simulink model "ADCS"  (R2024a)
settings: Solver=FixedStepDiscrete  StartTime=0.0  StopTime=86400  FixedStep=1  RelTol=1e-3  EnableMultiTasking=on
undefined symbols (not defined in the file): deg, rad, s
libraries: aerolibconvert2 x4, sharedtransform x3, aerolibutil x2
settings Model: Creator=Abhishek  LastModifiedBy=Abhishek
settings SolverCC: AutoInsertRateTranBlk=on

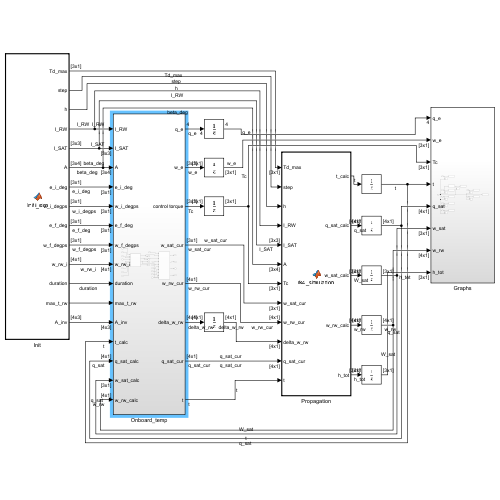
[thumbnail: Simulink's stored preview of the top-level diagram]
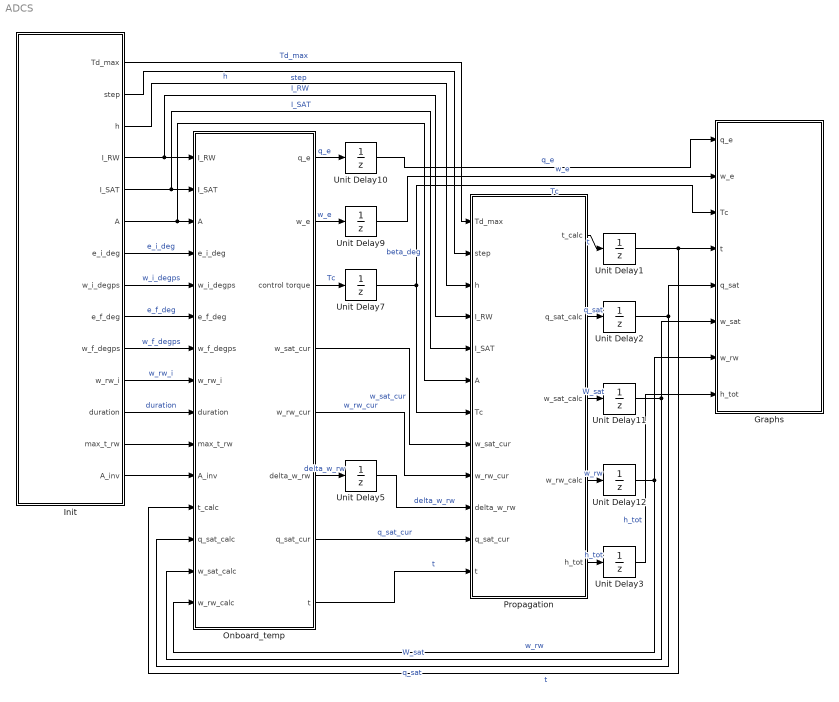
== system ADCS ==
  Graphs : Subsystem
  Init : MATLAB Function  TreatAsAtomicUnit=on
  Onboard_temp : Subsystem
  Propagation : MATLAB Function  TreatAsAtomicUnit=on
  Unit Delay{1..3,5,7,9..12} (9 alike) : UnitDelay  SampleTime=-1  HasFrameUpgradeWarning=on
  wires:
  Init/8(w_i_degps) -> Onboard_temp/5(w_i_degps)  "w_i_degps"
  Init/5(I_SAT) -> Onboard_temp/2(I_SAT), Propagation/5(I_SAT)  "I_SAT"
  Init/10(w_f_degps) -> Onboard_temp/7(w_f_degps)  "w_f_degps"
  Init/4(I_RW) -> Onboard_temp/1(I_RW), Propagation/4(I_RW)  "I_RW"
  Init/7(e_i_deg) -> Onboard_temp/4(e_i_deg)  "e_i_deg"
  Init/9(e_f_deg) -> Onboard_temp/6(e_f_deg)  "e_f_deg"
  Unit Delay11/1 -> Onboard_temp/14(w_sat_calc), Graphs/6(w_sat)  "W_sat"
  Init/2(step) -> Propagation/2(step)  "step"
  Init/11(w_rw_i) -> Onboard_temp/8(w_rw_i)  "w_rw_i"
  Init/3(h) -> Propagation/3(h)  "h"
  Init/12(duration) -> Onboard_temp/9(duration)  "duration"
  Unit Delay2/1 -> Onboard_temp/13(q_sat_calc), Graphs/5(q_sat)  "q_sat"
  Unit Delay9/1 -> Graphs/2(w_e)  "w_e"
  Init/6(A) -> Onboard_temp/3(A), Propagation/6(A)  "beta_deg"
  Unit Delay1/1 -> Graphs/4(t), Onboard_temp/12(t_calc)  "t"
  Init/1(Td_max) -> Propagation/1(Td_max)  "Td_max"
  Unit Delay7/1 -> Propagation/7(Tc), Graphs/3(Tc)  "Tc"
  Unit Delay10/1 -> Graphs/1(q_e)  "q_e"
  Unit Delay5/1 -> Propagation/10(delta_w_rw)  "delta_w_rw"
  Onboard_temp/8(t) -> Propagation/12(t)  "t"
  Onboard_temp/7(q_sat_cur) -> Propagation/11(q_sat_cur)  "q_sat_cur"
  Onboard_temp/6(delta_w_rw) -> Unit Delay5/1  "delta_w_rw"
  Onboard_temp/5(w_rw_cur) -> Propagation/9(w_rw_cur)  "w_rw_cur"
  Onboard_temp/3(control torque) -> Unit Delay7/1  "Tc"
  Onboard_temp/4(w_sat_cur) -> Propagation/8(w_sat_cur)  "w_sat_cur"
  Onboard_temp/2(w_e) -> Unit Delay9/1  "w_e"
  Onboard_temp/1(q_e) -> Unit Delay10/1  "q_e"
  Unit Delay12/1 -> Onboard_temp/15(w_rw_calc), Graphs/7(w_rw)  "w_rw"
  Propagation/1(t_calc) -> Unit Delay1/1  "t"
  Propagation/2(q_sat_calc) -> Unit Delay2/1  "q_sat"
  Propagation/3(w_sat_calc) -> Unit Delay11/1  "W_sat"
  Propagation/4(w_rw_calc) -> Unit Delay12/1  "w_rw"
  Init/14(A_inv) -> Onboard_temp/11(A_inv)
  Init/13(max_t_rw) -> Onboard_temp/10(max_t_rw)
  Unit Delay3/1 -> Graphs/8(h_tot)  "h_tot"
  Propagation/5(h_tot) -> Unit Delay3/1  "h_tot"

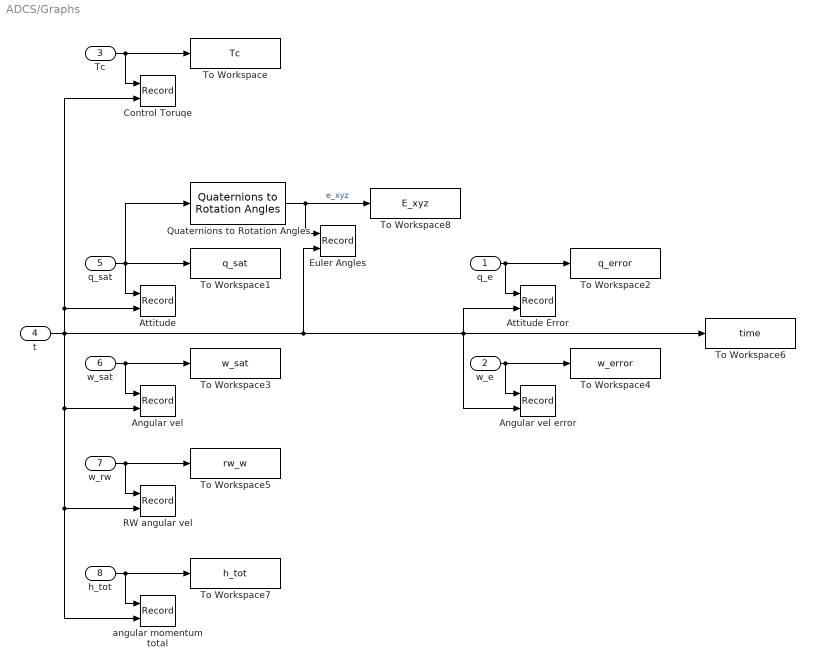
== system ADCS/Graphs ==
  q_e : Inport
  w_e : Inport  Port=2
  Tc : Inport  Port=3
  t : Inport  Port=4
  q_sat : Inport  Port=5
  w_sat : Inport  Port=6
  w_rw : Inport  Port=7
  h_tot : Inport  Port=8
  Angular vel : Record  FileSettingsInternal="{\"entries\":[{\"content\":{\"excelSettings\":{\"content\":{},\"type\":\"Streamout.ExcelSettings\"}},\"type\":\"Streamout.FileSettingStorage\",\"uuid\":\"\"}],\"packageUris\":[\"http:\\/\\/schema.mathworks.com\\/mf0\\/streamout_blocks\\/R2020a\"],\"version\":\"1.0\"}"  Layout=[1 1]  SignalsInternal="{\"entries\":[{\"content\":{\"signals\":[{\"content\":{\"blockPath\":[],\"dimensions\":[3,1],\"domain\":\"\",\"hasChildren\":true,\"lineColor\":\"#139fff\",\"lineWidth\":2,\"port\":1,\"sid\":[\"\"],\"signalID\":1,\"signalName\":\"w_sat\"},\"type\":\"RecordBlkView.Signal\",\"uuid\":\"\"},{\"content\":{\"blockPath\":[],\"channel\":[1,1],\"dimensions\":[3,1],\"domain\":\"\",\"lineColor\":\"#139fff\",\"lineWidth\":2,\"parentID\":1,\"plots\":[ 1 ],\"port\":1,\"sid\":[\"\"],\"signalID\":2,\"signalName\":\"w_sat\"},\"type\":\"RecordBlkView.Signal\",\"uuid\":\"\"},{\"content\":{\"blockPath\":[],\"dimensions\":[1],\"domain\":\"\",\"lineColor\":\"#ff6929\",\"lineWidth\":2,\"port\":2,\"sid\":[\"\"],\"signalID\":3,\"signalName\":\"t\"},\"type\":\"RecordBlkView.Signal\",\"uuid\":\"\"},{\"content\":{\"blockPath\":[],\"channel\":[2,1],\"dimensions\":[3,1],\"domain\":\"\",\"lineColor\":\"#4dbeee\",\"lineWidth\":2,\"parentID\":1,\"plots\":[ 1 ],\"port\":1,\"sid\":[\"\"],\"signalID\":4,\"signalName\":\"w_sat\"},\"type\":\"RecordBlkView.Signal\",\"uuid\":\"\"},{\"content\":{\"blockPath\":[],\"channel\":[3,1],\"dimensions\":[3,1],\"domain\":\"\",\"lineColor\":\"#a2142f\",\"lineWidth\":2,\"parentID\":1,\"plots\":[ 1 ],\"port\":1,\"sid\":[\"\"],\"signalID\":5,\"signalName\":\"w_sat\"},\"type\":\"RecordBlkView.Signal\",\"uuid\":\"\"}]},\"type\":\"RecordBlkView.InputSignals\",\"uuid\":\"\"}],\"packageUris\":[\"http:\\/\\/schema.mathworks.com\\/mf0\\/streamout_blocks\\/R2020a\"],\"version\":\"1.0\"}"  CompatibilityTag=XY
  Angular vel error : Record  FileSettingsInternal="{\"entries\":[{\"content\":{\"excelSettings\":{\"content\":{},\"type\":\"Streamout.ExcelSettings\"}},\"type\":\"Streamout.FileSettingStorage\",\"uuid\":\"\"}],\"packageUris\":[\"http:\\/\\/schema.mathworks.com\\/mf0\\/streamout_blocks\\/R2020a\"],\"version\":\"1.0\"}"  Layout=[1 1]  SignalsInternal="{\"entries\":[{\"content\":{\"signals\":[{\"content\":{\"blockPath\":[],\"dimensions\":[3,1],\"domain\":\"\",\"hasChildren\":true,\"lineColor\":\"#64d413\",\"lineWidth\":2,\"port\":1,\"sid\":[\"\"],\"signalID\":1,\"signalName\":\"w_e\"},\"type\":\"RecordBlkView.Signal\",\"uuid\":\"\"},{\"content\":{\"blockPath\":[],\"channel\":[1,1],\"dimensions\":[3,1],\"domain\":\"\",\"lineColor\":\"#64d413\",\"lineWidth\":2,\"parentID\":1,\"plots\":[ 1 ],\"port\":1,\"sid\":[\"\"],\"signalID\":2,\"signalName\":\"w_e\"},\"type\":\"RecordBlkView.Signal\",\"uuid\":\"\"},{\"content\":{\"blockPath\":[],\"dimensions\":[1],\"domain\":\"\",\"lineColor\":\"#ff13a6\",\"lineWidth\":2,\"port\":2,\"sid\":[\"\"],\"signalID\":3,\"signalName\":\"t\"},\"type\":\"RecordBlkView.Signal\",\"uuid\":\"\"},{\"content\":{\"blockPath\":[],\"channel\":[2,1],\"dimensions\":[3,1],\"domain\":\"\",\"lineColor\":\"#139fff\",\"lineWidth\":2,\"parentID\":1,\"plots\":[ 1 ],\"port\":1,\"sid\":[\"\"],\"signalID\":4,\"signalName\":\"w_e\"},\"type\":\"RecordBlkView.Signal\",\"uuid\":\"\"},{\"content\":{\"blockPath\":[],\"channel\":[3,1],\"dimensions\":[3,1],\"domain\":\"\",\"lineColor\":\"#ff6929\",\"lineWidth\":2,\"parentID\":1,\"plots\":[ 1 ],\"port\":1,\"sid\":[\"\"],\"signalID\":5,\"signalName\":\"w_e\"},\"type\":\"RecordBlkView.Signal\",\"uuid\":\"\"}]},\"type\":\"RecordBlkView.InputSignals\",\"uuid\":\"\"}],\"packageUris\":[\"http:\\/\\/schema.mathworks.com\\/mf0\\/streamout_blocks\\/R2020a\"],\"version\":\"1.0\"}"  CompatibilityTag=XY
  Attitude : Record  RecordToWorkspace=on  FileSettingsInternal="{\"entries\":[{\"content\":{\"excelSettings\":{\"content\":{},\"type\":\"Streamout.ExcelSettings\"}},\"type\":\"Streamout.FileSettingStorage\",\"uuid\":\"\"}],\"packageUris\":[\"http:\\/\\/schema.mathworks.com\\/mf0\\/streamout_blocks\\/R2020a\"],\"version\":\"1.0\"}"  Layout=[1 1]  SignalsInternal="{\"entries\":[{\"content\":{\"signals\":[{\"content\":{\"blockPath\":[],\"dimensions\":[4,1],\"domain\":\"\",\"hasChildren\":true,\"lineColor\":\"#22b573\",\"lineWidth\":2,\"port\":1,\"sid\":[\"\"],\"signalID\":1,\"signalName\":\"q_sat\"},\"type\":\"RecordBlkView.Signal\",\"uuid\":\"\"},{\"content\":{\"blockPath\":[],\"channel\":[1,1],\"dimensions\":[4,1],\"domain\":\"\",\"lineColor\":\"#22b573\",\"lineWidth\":2,\"parentID\":1,\"plots\":[ 1 ],\"port\":1,\"sid\":[\"\"],\"signalID\":2,\"signalName\":\"q_sat\"},\"type\":\"RecordBlkView.Signal\",\"uuid\":\"\"},{\"content\":{\"blockPath\":[],\"dimensions\":[1],\"domain\":\"\",\"lineColor\":\"#0072bd\",\"lineWidth\":2,\"port\":2,\"sid\":[\"\"],\"signalID\":3,\"signalName\":\"t\"},\"type\":\"RecordBlkView.Signal\",\"uuid\":\"\"},{\"content\":{\"blockPath\":[],\"channel\":[2,1],\"dimensions\":[4,1],\"domain\":\"\",\"lineColor\":\"#b746ff\",\"lineWidth\":2,\"parentID\":1,\"plots\":[ 1 ],\"port\":1,\"sid\":[\"\"],\"signalID\":4,\"signalName\":\"q_sat\"},\"type\":\"RecordBlkView.Signal\",\"uuid\":\"\"},{\"content\":{\"blockPath\":[],\"channel\":[3,1],\"dimensions\":[4,1],\"domain\":\"\",\"lineColor\":\"#64d413\",\"lineWidth\":2,\"parentID\":1,\"plots\":[ 1 ],\"port\":1,\"sid\":[\"\"],\"signalID\":5,\"signalName\":\"q_sat\"},\"type\":\"RecordBlkView.Signal\",\"uuid\":\"\"},{\"content\":{\"blockPath\":[],\"channel\":[4,1],\"dimensions\":[4,1],\"domain\":\"\",\"lineColor\":\"#ff13a6\",\"lineWidth\":2,\"parentID\":1,\"plots\":[ 1 ],\"port\":1,\"sid\":[\"\"],\"signalID\":6,\"signalName\":\"q_sat\"},\"type\":\"RecordBlkView.Signal\",\"uuid\":\"\"}]},\"type\":\"RecordBlkView.InputSignals\",\"uuid\":\"\"}],\"packageUris\":[\"http:\\/\\/schema.mathworks.com\\/mf0\\/streamout_blocks\\/R2020a\"],\"version\":\"1.0\"}"  CompatibilityTag=XY
  Attitude Error : Record  FileSettingsInternal="{\"entries\":[{\"content\":{\"excelSettings\":{\"content\":{},\"type\":\"Streamout.ExcelSettings\"}},\"type\":\"Streamout.FileSettingStorage\",\"uuid\":\"\"}],\"packageUris\":[\"http:\\/\\/schema.mathworks.com\\/mf0\\/streamout_blocks\\/R2020a\"],\"version\":\"1.0\"}"  Layout=[1 1]  SignalsInternal="{\"entries\":[{\"content\":{\"signals\":[{\"content\":{\"blockPath\":[],\"dimensions\":[4],\"domain\":\"\",\"hasChildren\":true,\"lineColor\":\"#edb120\",\"lineWidth\":2,\"port\":1,\"sid\":[\"\"],\"signalID\":1,\"signalName\":\"q_e\"},\"type\":\"RecordBlkView.Signal\",\"uuid\":\"\"},{\"content\":{\"blockPath\":[],\"channel\":[1],\"dimensions\":[4],\"domain\":\"\",\"lineColor\":\"#edb120\",\"lineWidth\":2,\"parentID\":1,\"plots\":[ 1 ],\"port\":1,\"sid\":[\"\"],\"signalID\":2,\"signalName\":\"q_e\"},\"type\":\"RecordBlkView.Signal\",\"uuid\":\"\"},{\"content\":{\"blockPath\":[],\"dimensions\":[1],\"domain\":\"\",\"lineColor\":\"#7e2f8e\",\"lineWidth\":2,\"port\":2,\"sid\":[\"\"],\"signalID\":3,\"signalName\":\"t\"},\"type\":\"RecordBlkView.Signal\",\"uuid\":\"\"},{\"content\":{\"blockPath\":[],\"channel\":[2],\"dimensions\":[4],\"domain\":\"\",\"lineColor\":\"#fe330a\",\"lineWidth\":2,\"parentID\":1,\"plots\":[ 1 ],\"port\":1,\"sid\":[\"\"],\"signalID\":4,\"signalName\":\"q_e\"},\"type\":\"RecordBlkView.Signal\",\"uuid\":\"\"},{\"content\":{\"blockPath\":[],\"channel\":[3],\"dimensions\":[4],\"domain\":\"\",\"lineColor\":\"#22b573\",\"lineWidth\":2,\"parentID\":1,\"plots\":[ 1 ],\"port\":1,\"sid\":[\"\"],\"signalID\":5,\"signalName\":\"q_e\"},\"type\":\"RecordBlkView.Signal\",\"uuid\":\"\"},{\"content\":{\"blockPath\":[],\"channel\":[4],\"dimensions\":[4],\"domain\":\"\",\"lineColor\":\"#0072bd\",\"lineWidth\":2,\"parentID\":1,\"plots\":[ 1 ],\"port\":1,\"sid\":[\"\"],\"signalID\":6,\"signalName\":\"q_e\"},\"type\":\"RecordBlkView.Signal\",\"uuid\":\"\"}]},\"type\":\"RecordBlkView.InputSignals\",\"uuid\":\"\"}],\"packageUris\":[\"http:\\/\\/schema.mathworks.com\\/mf0\\/streamout_blocks\\/R2020a\"],\"version\":\"1.0\"}"  CompatibilityTag=XY
  Control Toruqe : Record  FileSettingsInternal="{\"entries\":[{\"content\":{\"excelSettings\":{\"content\":{},\"type\":\"Streamout.ExcelSettings\"}},\"type\":\"Streamout.FileSettingStorage\",\"uuid\":\"\"}],\"packageUris\":[\"http:\\/\\/schema.mathworks.com\\/mf0\\/streamout_blocks\\/R2020a\"],\"version\":\"1.0\"}"  Layout=[1 1]  SignalsInternal="{\"entries\":[{\"content\":{\"signals\":[{\"content\":{\"blockPath\":[],\"dimensions\":[3,1],\"domain\":\"\",\"hasChildren\":true,\"lineColor\":\"#4dbeee\",\"lineWidth\":2,\"port\":1,\"sid\":[\"\"],\"signalID\":1,\"signalName\":\"Tc\"},\"type\":\"RecordBlkView.Signal\",\"uuid\":\"\"},{\"content\":{\"blockPath\":[],\"channel\":[1,1],\"dimensions\":[3,1],\"domain\":\"\",\"lineColor\":\"#4dbeee\",\"lineWidth\":2,\"parentID\":1,\"plots\":[ 1 ],\"port\":1,\"sid\":[\"\"],\"signalID\":2,\"signalName\":\"Tc\"},\"type\":\"RecordBlkView.Signal\",\"uuid\":\"\"},{\"content\":{\"blockPath\":[],\"dimensions\":[1],\"domain\":\"\",\"lineColor\":\"#a2142f\",\"lineWidth\":2,\"port\":2,\"sid\":[\"\"],\"signalID\":3,\"signalName\":\"t\"},\"type\":\"RecordBlkView.Signal\",\"uuid\":\"\"},{\"content\":{\"blockPath\":[],\"channel\":[2,1],\"dimensions\":[3,1],\"domain\":\"\",\"lineColor\":\"#d95319\",\"lineWidth\":2,\"parentID\":1,\"plots\":[ 1 ],\"port\":1,\"sid\":[\"\"],\"signalID\":4,\"signalName\":\"Tc\"},\"type\":\"RecordBlkView.Signal\",\"uuid\":\"\"},{\"content\":{\"blockPath\":[],\"channel\":[3,1],\"dimensions\":[3,1],\"domain\":\"\",\"lineColor\":\"#edb120\",\"lineWidth\":2,\"parentID\":1,\"plots\":[ 1 ],\"port\":1,\"sid\":[\"\"],\"signalID\":5,\"signalName\":\"Tc\"},\"type\":\"RecordBlkView.Signal\",\"uuid\":\"\"}]},\"type\":\"RecordBlkView.InputSignals\",\"uuid\":\"\"}],\"packageUris\":[\"http:\\/\\/schema.mathworks.com\\/mf0\\/streamout_blocks\\/R2020a\"],\"version\":\"1.0\"}"  CompatibilityTag=XY
  Euler Angles : Record  FileSettingsInternal="{\"entries\":[{\"content\":{\"excelSettings\":{\"content\":{},\"type\":\"Streamout.ExcelSettings\"}},\"type\":\"Streamout.FileSettingStorage\",\"uuid\":\"\"}],\"packageUris\":[\"http:\\/\\/schema.mathworks.com\\/mf0\\/streamout_blocks\\/R2020a\"],\"version\":\"1.0\"}"  Layout=[1 1]  SignalsInternal="{\"entries\":[{\"content\":{\"signals\":[{\"content\":{\"blockPath\":[],\"dimensions\":[3],\"domain\":\"\",\"hasChildren\":true,\"lineColor\":\"#ff6929\",\"lineWidth\":2,\"port\":1,\"sid\":[\"\"],\"signalID\":1,\"signalName\":\"e_xyz\"},\"type\":\"RecordBlkView.Signal\",\"uuid\":\"\"},{\"content\":{\"blockPath\":[],\"channel\":[1],\"dimensions\":[3],\"domain\":\"\",\"lineColor\":\"#ff6929\",\"lineWidth\":2,\"parentID\":1,\"plots\":[ 1 ],\"port\":1,\"sid\":[\"\"],\"signalID\":2,\"signalName\":\"e_xyz\"},\"type\":\"RecordBlkView.Signal\",\"uuid\":\"\"},{\"content\":{\"blockPath\":[],\"dimensions\":[1],\"domain\":\"\",\"lineColor\":\"#b746ff\",\"lineWidth\":2,\"port\":2,\"sid\":[\"\"],\"signalID\":3,\"signalName\":\"t\"},\"type\":\"RecordBlkView.Signal\",\"uuid\":\"\"},{\"content\":{\"blockPath\":[],\"channel\":[2],\"dimensions\":[3],\"domain\":\"\",\"lineColor\":\"#7e2f8e\",\"lineWidth\":2,\"parentID\":1,\"plots\":[ 1 ],\"port\":1,\"sid\":[\"\"],\"signalID\":4,\"signalName\":\"e_xyz\"},\"type\":\"RecordBlkView.Signal\",\"uuid\":\"\"},{\"content\":{\"blockPath\":[],\"channel\":[3],\"dimensions\":[3],\"domain\":\"\",\"lineColor\":\"#77ac30\",\"lineWidth\":2,\"parentID\":1,\"plots\":[ 1 ],\"port\":1,\"sid\":[\"\"],\"signalID\":5,\"signalName\":\"e_xyz\"},\"type\":\"RecordBlkView.Signal\",\"uuid\":\"\"}]},\"type\":\"RecordBlkView.InputSignals\",\"uuid\":\"\"}],\"packageUris\":[\"http:\\/\\/schema.mathworks.com\\/mf0\\/streamout_blocks\\/R2020a\"],\"version\":\"1.0\"}"  CompatibilityTag=XY
  Quaternions to Rotation Angles : sharedtransform/Quaternions to Rotation Angles  rotationOrder=XYZ  aMode=aMode
  RW angular vel : Record  FileSettingsInternal="{\"entries\":[{\"content\":{\"excelSettings\":{\"content\":{},\"type\":\"Streamout.ExcelSettings\"}},\"type\":\"Streamout.FileSettingStorage\",\"uuid\":\"\"}],\"packageUris\":[\"http:\\/\\/schema.mathworks.com\\/mf0\\/streamout_blocks\\/R2020a\"],\"version\":\"1.0\"}"  Layout=[1 1]  SignalsInternal="{\"entries\":[{\"content\":{\"signals\":[{\"content\":{\"blockPath\":[],\"dimensions\":[4,1],\"domain\":\"\",\"hasChildren\":true,\"lineColor\":\"#ff13a6\",\"lineWidth\":2,\"port\":1,\"sid\":[\"\"],\"signalID\":1,\"signalName\":\"w_rw\"},\"type\":\"RecordBlkView.Signal\",\"uuid\":\"\"},{\"content\":{\"blockPath\":[],\"channel\":[1,1],\"dimensions\":[4,1],\"domain\":\"\",\"lineColor\":\"#ff13a6\",\"lineWidth\":2,\"parentID\":1,\"plots\":[ 1 ],\"port\":1,\"sid\":[\"\"],\"signalID\":2,\"signalName\":\"w_rw\"},\"type\":\"RecordBlkView.Signal\",\"uuid\":\"\"},{\"content\":{\"blockPath\":[],\"dimensions\":[1],\"domain\":\"\",\"lineColor\":\"#fe330a\",\"lineWidth\":2,\"port\":2,\"sid\":[\"\"],\"signalID\":3,\"signalName\":\"t\"},\"type\":\"RecordBlkView.Signal\",\"uuid\":\"\"},{\"content\":{\"blockPath\":[],\"channel\":[2,1],\"dimensions\":[4,1],\"domain\":\"\",\"lineColor\":\"#4dbeee\",\"lineWidth\":2,\"parentID\":1,\"plots\":[ 1 ],\"port\":1,\"sid\":[\"\"],\"signalID\":4,\"signalName\":\"w_rw\"},\"type\":\"RecordBlkView.Signal\",\"uuid\":\"\"},{\"content\":{\"blockPath\":[],\"channel\":[3,1],\"dimensions\":[4,1],\"domain\":\"\",\"lineColor\":\"#a2142f\",\"lineWidth\":2,\"parentID\":1,\"plots\":[ 1 ],\"port\":1,\"sid\":[\"\"],\"signalID\":5,\"signalName\":\"w_rw\"},\"type\":\"RecordBlkView.Signal\",\"uuid\":\"\"},{\"content\":{\"blockPath\":[],\"channel\":[4,1],\"dimensions\":[4,1],\"domain\":\"\",\"lineColor\":\"#139fff\",\"lineWidth\":2,\"parentID\":1,\"plots\":[ 1 ],\"port\":1,\"sid\":[\"\"],\"signalID\":6,\"signalName\":\"w_rw\"},\"type\":\"RecordBlkView.Signal\",\"uuid\":\"\"}]},\"type\":\"RecordBlkView.InputSignals\",\"uuid\":\"\"}],\"packageUris\":[\"http:\\/\\/schema.mathworks.com\\/mf0\\/streamout_blocks\\/R2020a\"],\"version\":\"1.0\"}"  CompatibilityTag=XY
  To Workspace : ToWorkspace  VariableName=Tc  SampleTime=-1
  To Workspace1 : ToWorkspace  VariableName=q_sat  SampleTime=-1
  To Workspace2 : ToWorkspace  VariableName=q_error  SampleTime=-1
  To Workspace3 : ToWorkspace  VariableName=w_sat  SampleTime=-1
  To Workspace4 : ToWorkspace  VariableName=w_error  SampleTime=-1
  To Workspace5 : ToWorkspace  VariableName=rw_w  SampleTime=-1
  To Workspace6 : ToWorkspace  VariableName=time  SampleTime=-1
  To Workspace7 : ToWorkspace  VariableName=h_tot  SampleTime=-1
  To Workspace8 : ToWorkspace  VariableName=E_xyz  SampleTime=-1
  angular momentum total : Record  FileSettingsInternal="{\"entries\":[{\"content\":{\"excelSettings\":{\"content\":{},\"type\":\"Streamout.ExcelSettings\"}},\"type\":\"Streamout.FileSettingStorage\",\"uuid\":\"\"}],\"packageUris\":[\"http:\\/\\/schema.mathworks.com\\/mf0\\/streamout_blocks\\/R2020a\"],\"version\":\"1.0\"}"  Layout=[1 1]  SignalsInternal="{\"entries\":[{\"content\":{\"signals\":[{\"content\":{\"blockPath\":[],\"dimensions\":[3,1],\"domain\":\"\",\"hasChildren\":true,\"lineColor\":\"#7e2f8e\",\"lineWidth\":2,\"port\":1,\"sid\":[\"\"],\"signalID\":1,\"signalName\":\"h_tot\"},\"type\":\"RecordBlkView.Signal\",\"uuid\":\"\"},{\"content\":{\"blockPath\":[],\"channel\":[1,1],\"dimensions\":[3,1],\"domain\":\"\",\"lineColor\":\"#7e2f8e\",\"lineWidth\":2,\"parentID\":1,\"plots\":[ 1 ],\"port\":1,\"sid\":[\"\"],\"signalID\":2,\"signalName\":\"h_tot\"},\"type\":\"RecordBlkView.Signal\",\"uuid\":\"\"},{\"content\":{\"blockPath\":[],\"dimensions\":[1],\"domain\":\"\",\"lineColor\":\"#77ac30\",\"lineWidth\":2,\"port\":2,\"sid\":[\"\"],\"signalID\":3,\"signalName\":\"t\"},\"type\":\"RecordBlkView.Signal\",\"uuid\":\"\"},{\"content\":{\"blockPath\":[],\"channel\":[2,1],\"dimensions\":[3,1],\"domain\":\"\",\"lineColor\":\"#22b573\",\"lineWidth\":2,\"parentID\":1,\"plots\":[ 1 ],\"port\":1,\"sid\":[\"\"],\"signalID\":4,\"signalName\":\"h_tot\"},\"type\":\"RecordBlkView.Signal\",\"uuid\":\"\"},{\"content\":{\"blockPath\":[],\"channel\":[3,1],\"dimensions\":[3,1],\"domain\":\"\",\"lineColor\":\"#0072bd\",\"lineWidth\":2,\"parentID\":1,\"plots\":[ 1 ],\"port\":1,\"sid\":[\"\"],\"signalID\":5,\"signalName\":\"h_tot\"},\"type\":\"RecordBlkView.Signal\",\"uuid\":\"\"}]},\"type\":\"RecordBlkView.InputSignals\",\"uuid\":\"\"}],\"packageUris\":[\"http:\\/\\/schema.mathworks.com\\/mf0\\/streamout_blocks\\/R2020a\"],\"version\":\"1.0\"}"  VisualizationBindings="{\"sparklinesplugin\":{\"info\":[{\"bindingParametersList\":[],\"subplotID\":1}]}}"  CompatibilityTag=XY
  wires:
  w_sat/1 -> To Workspace3/1, Angular vel/1
  q_e/1 -> Attitude Error/1, To Workspace2/1
  q_sat/1 -> To Workspace1/1, Quaternions to Rotation Angles/1, Attitude/1
  w_e/1 -> To Workspace4/1, Angular vel error/1
  Tc/1 -> To Workspace/1, Control Toruqe/1
  w_rw/1 -> RW angular vel/1, To Workspace5/1
  t/1 -> Euler Angles/2, To Workspace6/1, Attitude Error/2, Angular vel error/2, Angular vel/2, angular momentum total/2, RW angular vel/2, Attitude/2, Control Toruqe/2
  h_tot/1 -> To Workspace7/1, angular momentum total/1
  Quaternions to Rotation Angles/1 -> To Workspace8/1, Euler Angles/1  "e_xyz"

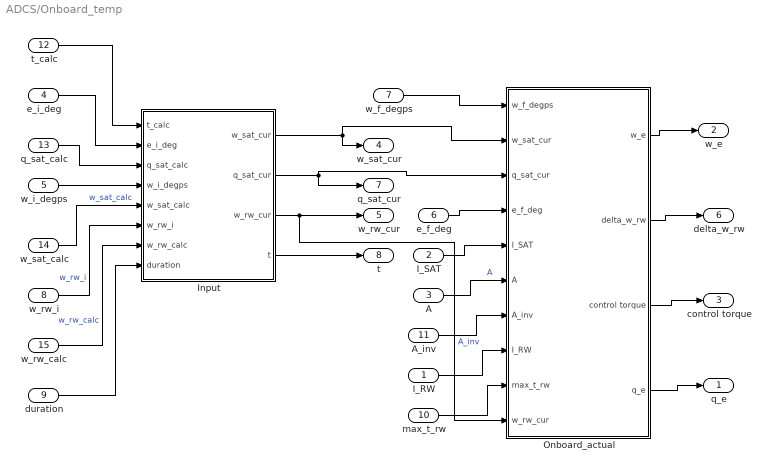
== system ADCS/Onboard_temp ==
  I_RW : Inport
  I_SAT : Inport  Port=2
  A : Inport  Port=3
  e_i_deg : Inport  Port=4
  w_i_degps : Inport  Port=5
  e_f_deg : Inport  Port=6
  w_f_degps : Inport  Port=7
  w_rw_i : Inport  Port=8
  duration : Inport  Port=9
  max_t_rw : Inport  Port=10
  A_inv : Inport  Port=11
  t_calc : Inport  Port=12
  q_sat_calc : Inport  Port=13
  w_sat_calc : Inport  Port=14
  w_rw_calc : Inport  Port=15
  Input : Subsystem
  Onboard_actual : Subsystem
  q_e : Outport
  w_e : Outport  Port=2
  control torque : Outport  Port=3
  w_sat_cur : Outport  Port=4
  w_rw_cur : Outport  Port=5
  delta_w_rw : Outport  Port=6
  q_sat_cur : Outport  Port=7
  t : Outport  Port=8
  wires:
  w_rw_i/1 -> Input/6(w_rw_i)  "w_rw_i"
  duration/1 -> Input/8(duration)
  Input/3(w_rw_cur) -> Onboard_actual/10(w_rw_cur), w_rw_cur/1
  w_rw_calc/1 -> Input/7(w_rw_calc)  "w_rw_calc"
  t_calc/1 -> Input/1(t_calc)
  Onboard_actual/1(w_e) -> w_e/1
  e_i_deg/1 -> Input/2(e_i_deg)
  q_sat_calc/1 -> Input/3(q_sat_calc)
  w_i_degps/1 -> Input/4(w_i_degps)
  w_sat_calc/1 -> Input/5(w_sat_calc)  "w_sat_calc"
  Input/1(w_sat_cur) -> w_sat_cur/1, Onboard_actual/2(w_sat_cur)
  Onboard_actual/3(control torque) -> control torque/1
  Input/2(q_sat_cur) -> q_sat_cur/1, Onboard_actual/3(q_sat_cur)
  Input/4(t) -> t/1
  w_f_degps/1 -> Onboard_actual/1(w_f_degps)
  e_f_deg/1 -> Onboard_actual/4(e_f_deg)
  I_SAT/1 -> Onboard_actual/5(I_SAT)
  Onboard_actual/2(delta_w_rw) -> delta_w_rw/1
  Onboard_actual/4(q_e) -> q_e/1
  A/1 -> Onboard_actual/6(A)  "A"
  I_RW/1 -> Onboard_actual/8(I_RW)
  A_inv/1 -> Onboard_actual/7(A_inv)  "A_inv"
  max_t_rw/1 -> Onboard_actual/9(max_t_rw)

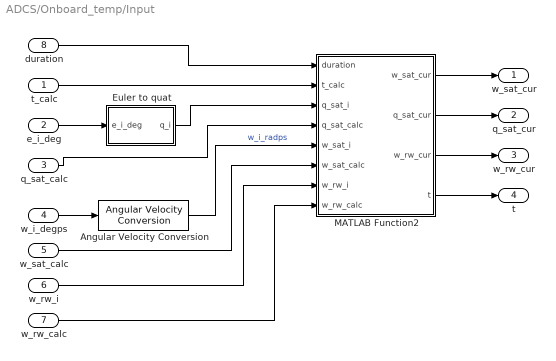
== system ADCS/Onboard_temp/Input ==
  t_calc : Inport
  e_i_deg : Inport  Port=2
  q_sat_calc : Inport  Port=3
  w_i_degps : Inport  Port=4
  w_sat_calc : Inport  Port=5
  w_rw_i : Inport  Port=6
  w_rw_calc : Inport  Port=7
  duration : Inport  Port=8
  Angular Velocity Conversion : aerolibconvert2/Angular Velocity Conversion  IU=deg/s  OU=rad/s
  Euler to quat : Subsystem
  MATLAB Function2 : MATLAB Function  TreatAsAtomicUnit=on
  w_sat_cur : Outport
  q_sat_cur : Outport  Port=2
  w_rw_cur : Outport  Port=3
  t : Outport  Port=4
  wires:
  MATLAB Function2/3(w_rw_cur) -> w_rw_cur/1
  Angular Velocity Conversion/1 -> MATLAB Function2/5(w_sat_i)  "w_i_radps"
  w_rw_calc/1 -> MATLAB Function2/8(w_rw_calc)
  MATLAB Function2/2(q_sat_cur) -> q_sat_cur/1
  Euler to quat/1(q_i) -> MATLAB Function2/3(q_sat_i)
  t_calc/1 -> MATLAB Function2/2(t_calc)
  w_i_degps/1 -> Angular Velocity Conversion/1
  q_sat_calc/1 -> MATLAB Function2/4(q_sat_calc)
  w_sat_calc/1 -> MATLAB Function2/6(w_sat_calc)
  w_rw_i/1 -> MATLAB Function2/7(w_rw_i)
  MATLAB Function2/4(t) -> t/1
  e_i_deg/1 -> Euler to quat/1(e_i_deg)
  MATLAB Function2/1(w_sat_cur) -> w_sat_cur/1
  duration/1 -> MATLAB Function2/1(duration)

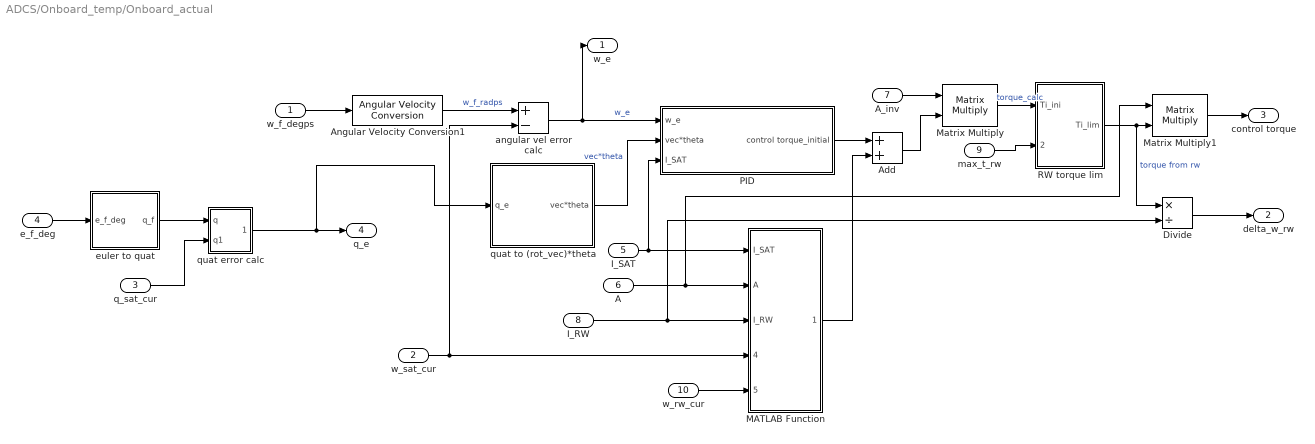
== system ADCS/Onboard_temp/Onboard_actual ==
  w_f_degps : Inport
  w_sat_cur : Inport  Port=2
  q_sat_cur : Inport  Port=3
  e_f_deg : Inport  Port=4
  I_SAT : Inport  Port=5
  A : Inport  Port=6
  A_inv : Inport  Port=7
  I_RW : Inport  Port=8
  max_t_rw : Inport  Port=9
  w_rw_cur : Inport  Port=10
  Add : Sum
  Angular Velocity Conversion1 : aerolibconvert2/Angular Velocity Conversion  IU=deg/s  OU=rad/s
  Divide : Product  Inputs=*/
  MATLAB Function : MATLAB Function  TreatAsAtomicUnit=on
  Matrix Multiply : Product  Multiplication=Matrix(*)
  Matrix Multiply1 : Product  Multiplication=Matrix(*)
  PID : Subsystem
  RW torque lim : MATLAB Function  TreatAsAtomicUnit=on
  angular vel error calc : Sum  Inputs=+-
  euler to quat : Subsystem
  quat error calc : Subsystem
  "quat to (rot_vec)*theta " : Subsystem
  w_e : Outport
  delta_w_rw : Outport  Port=2
  control torque : Outport  Port=3
  q_e : Outport  Port=4
  wires:
  Angular Velocity Conversion1/1 -> angular vel error calc/1  "w_f_radps"
  A_inv/1 -> Matrix Multiply/1
  q_sat_cur/1 -> quat error calc/2(q1)
  I_RW/1 -> MATLAB Function/3(I_RW), Divide/2
  e_f_deg/1 -> euler to quat/1(e_f_deg)
  quat error calc/1(q_e) -> "quat to (rot_vec)*theta "/1(q_e), q_e/1
  "quat to (rot_vec)*theta "/1(vec*theta) -> PID/2(vec*theta)  "vec*theta"
  w_sat_cur/1 -> MATLAB Function/4(w_sat_cur), angular vel error calc/2
  w_f_degps/1 -> Angular Velocity Conversion1/1
  angular vel error calc/1 -> w_e/1, PID/1(w_e)  "w_e"
  euler to quat/1(q_f) -> quat error calc/1(q)
  max_t_rw/1 -> RW torque lim/2(max_t_rw)
  I_SAT/1 -> MATLAB Function/1(I_SAT), PID/3(I_SAT)
  A/1 -> Matrix Multiply1/1, MATLAB Function/2(A)
  PID/1(control torque_initial) -> Add/1
  w_rw_cur/1 -> MATLAB Function/5(w_rw_cur)
  MATLAB Function/1(offset_Tc) -> Add/2
  Add/1 -> Matrix Multiply/2
  Matrix Multiply/1 -> RW torque lim/1(Ti_ini)  "torque_calc"
  RW torque lim/1(Ti_lim) -> Divide/1, Matrix Multiply1/2  "torque from rw"
  Matrix Multiply1/1 -> control torque/1
  Divide/1 -> delta_w_rw/1

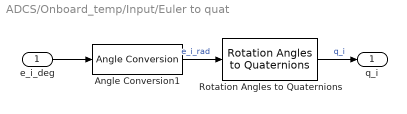
== system ADCS/Onboard_temp/Input/Euler to quat ==
  e_i_deg : Inport
  Angle Conversion1 : aerolibconvert2/Angle Conversion  IU=deg  OU=rad
  Rotation Angles to Quaternions : sharedtransform/Rotation Angles to Quaternions  rotationOrder=XYZ  aMode=aMode
  q_i : Outport
  wires:
  e_i_deg/1 -> Angle Conversion1/1
  Rotation Angles to Quaternions/1 -> q_i/1  "q_i"
  Angle Conversion1/1 -> Rotation Angles to Quaternions/1  "e_i_rad"

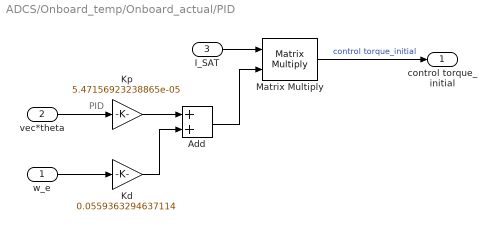
== system ADCS/Onboard_temp/Onboard_actual/PID ==
  note: PID
  w_e : Inport
  vec*theta : Inport  Port=2
  I_SAT : Inport  Port=3
  Add : Sum
  Kd : Gain  Gain=0.0559363294637114
  Kp : Gain  Gain=5.47156923238865e-05
  Matrix Multiply : Product  Multiplication=Matrix(*)
  control torque_initial : Outport
  wires:
  Matrix Multiply/1 -> control torque_initial/1  "control torque_initial"
  Kd/1 -> Add/2
  Kp/1 -> Add/1
  I_SAT/1 -> Matrix Multiply/1
  w_e/1 -> Kd/1
  vec*theta/1 -> Kp/1
  Add/1 -> Matrix Multiply/2

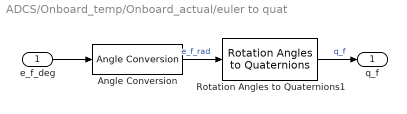
== system ADCS/Onboard_temp/Onboard_actual/euler to quat ==
  e_f_deg : Inport
  Angle Conversion : aerolibconvert2/Angle Conversion  IU=deg  OU=rad
  Rotation Angles to Quaternions1 : sharedtransform/Rotation Angles to Quaternions  rotationOrder=XYZ  aMode=aMode
  q_f : Outport
  wires:
  e_f_deg/1 -> Angle Conversion/1
  Angle Conversion/1 -> Rotation Angles to Quaternions1/1  "e_f_rad"
  Rotation Angles to Quaternions1/1 -> q_f/1  "q_f"

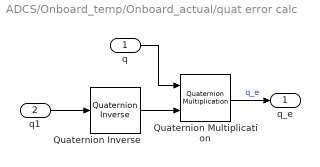
== system ADCS/Onboard_temp/Onboard_actual/quat error calc ==
  q : Inport
  q1 : Inport  Port=2
  Quaternion Inverse : aerolibutil/Quaternion Inverse
  Quaternion Multiplication : aerolibutil/Quaternion Multiplication
  q_e : Outport
  wires:
  q/1 -> Quaternion Multiplication/1
  q1/1 -> Quaternion Inverse/1
  Quaternion Multiplication/1 -> q_e/1  "q_e"
  Quaternion Inverse/1 -> Quaternion Multiplication/2

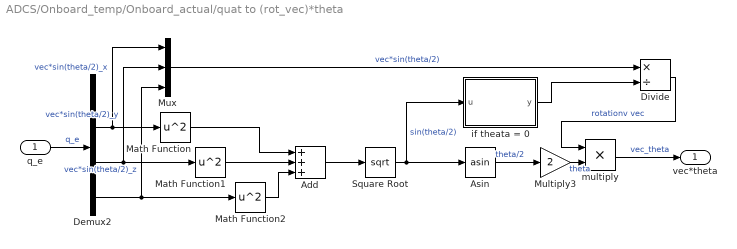
== system ADCS/Onboard_temp/Onboard_actual/quat to (rot_vec)*theta  ==
  q_e : Inport
  Add : Sum  Inputs=+++
  Asin : Trigonometry  Operator=asin
  Demux2 : Demux
  Divide : Product  Inputs=*/
  Math Function : Math  Operator=square
  Math Function1 : Math  Operator=square
  Math Function2 : Math  Operator=square
  Multiply3 : Gain  Gain=2
  Mux : Mux  Inputs=3
  Square Root : Sqrt
  if theata = 0 : MATLAB Function  TreatAsAtomicUnit=on
  multiply : Product  Inputs=**
  vec*theta : Outport
  wires:
  Demux2/2 -> Math Function/1, Mux/1  "vec*sin(theta/2)_x"
  Math Function2/1 -> Add/3
  Demux2/3 -> Math Function1/1, Mux/2  "vec*sin(theta/2)_y"
  Demux2/4 -> Math Function2/1, Mux/3  "vec*sin(theta/2)_z"
  Math Function1/1 -> Add/2
  q_e/1 -> Demux2/1  "q_e"
  Math Function/1 -> Add/1
  Add/1 -> Square Root/1
  Square Root/1 -> if theata = 0/1(u), Asin/1  "sin(theta/2)"
  Divide/1 -> multiply/1  "rotationv vec"
  Asin/1 -> Multiply3/1  "theta/2"
  Multiply3/1 -> multiply/2  "theta"
  multiply/1 -> vec*theta/1  "vec_theta"
  Mux/1 -> Divide/1  "vec*sin(theta/2)"
  if theata = 0/1(y) -> Divide/2

== matlab function ADCS/Onboard_temp/Onboard_actual/quat to (rot_vec)*theta /if theata = 0 ==
  data: u input; y output
function y = checking_zero(u)
    y=u;
    if u==0.00;
        y=1.00;
    end
end

== matlab function ADCS/Onboard_temp/Onboard_actual/MATLAB Function ==
  data: I_SAT input; A input; offset_Tc output; I_RW input; w_sat_cur input; w_rw_cur input
function offset_Tc = fcn(I_SAT,A,I_RW,w_sat_cur, w_rw_cur)
    offset_Tc=[0;0;0];
    H_sat= I_SAT*w_sat_cur;
    H_rw= A*(I_RW*w_rw_cur);
    offset_Tc=cross(w_sat_cur,H_sat)+cross(w_sat_cur,H_rw); 
end

== matlab function ADCS/Init ==
  data: Td_max output; step output; h output; I_RW output; I_SAT output; A output; e_i_deg output; w_i_degps output; e_f_deg output; w_f_degps output; w_rw_i output; duration output; max_t_rw output; A_inv output
function [Td_max,step,h,I_RW, I_SAT,A,e_i_deg,w_i_degps,e_f_deg,w_f_degps,w_rw_i,duration,max_t_rw,A_inv]= Initi_sim

    %beta_angle_deg=30; %Beta Angle of reaction wheels in Degrees 
    beta_angle_rad=asin(0.25); %Beta Angle of reaction wheels in Radians
    cB=cos(beta_angle_rad); %cos(beta)
    sB=sin(beta_angle_rad);%sin(beta)
    A=[cB, 0, -cB, 0; 0, cB, 0,-cB; sB, sB, sB, sB]; % Tc=A*Ti, where Tc is control torque (pid), Ti is torque by individual reaction wheels
    A_inv= pinv(A); %pseudo inverse of A

    e_f_deg=[30.00;50.00;70.00]; %Euler angles in degrees of final attitiude (XYZ)
    e_i_deg=[0.00;0.00;0.00]; %Euler angles in degrees of initial attitiude (XYZ)
    w_f_degps=[0;0;0];%[0.2;0.2;0.2]; % Final angular vel of satellite (deg/s)
    w_i_degps=[15.00;-15.00;15.00];% Initial Angular vel of satellite (deg/s)
    I_SAT=[2.10 0.00 0.01;0.00 2.30 -0.03;0.01 -0.03 1.72]; %Moment of Inertia of satellite
    I_RW=0.00042; %Moment of inertia of individual reaction wheels
    Td_max=[10.00^(-6);10.00^(-6);10.00^(-6)]; %max disturbance torque in Nm
    step=1; %step size of control loop in seconds
    H_rw_i=0.035;%Angular momentum of individual reaction wheel (Nms)
    w_rw_i=(H_rw_i/I_RW)*[1.00;1.00;1.00;1.00]; %initial angular vel of reaction wheels (rad/s)
    h=0.00125; %step size of propogation (angular vel and quaternions)
    duration=86400.0000; %duration of simulation in seconds
    max_t_rw=0.015; %max torque per reaction wheel Nm
end

== matlab function ADCS/Propagation ==
  data: Td_max input; step input; h input; I_RW input; I_SAT input; A input; Tc input; w_sat_cur input; w_rw_cur input; delta_w_rw input; q_sat_cur input; t input; t_calc output; q_sat_calc output; w_sat_calc output; w_rw_calc output; h_tot output
function [t_calc,q_sat_calc, w_sat_calc, w_rw_calc, h_tot] = rk4_simulation(Td_max,step, h,I_RW,I_SAT,A,Tc, w_sat_cur, w_rw_cur, delta_w_rw,q_sat_cur,t)
    Iinv=pinv(I_SAT); %inverse of Moment of inertia of satellite
    flag=0; %to toggle between initialized and calucated values in functions, had to do it some sort of complilation error.

    t_calc=-5.00; %initialzed time output to negative, just a sanity check to make sure the ouput of this funtion only goes into pid if initializations are done right
    
    %output initialized, compilation error
    h_rw_calc=[0.00;0.00;0.00];
    h_sat_calc=[0.00;0.00;0.00];
    h_tot=[0.00;0.00;0.00];

    q_sat_calc=[1;0;0;0]; %attitude of satellite 
    w_sat_calc=[0;0;0]; %angular vel of satellite (rad/s)
    w_rw_calc=[0;0;0;0]; %angular vel of reaction wheel (rad/s)
    h_rw_cur=[0.00;0.00;0.00]; %current angular momentum of reaction wheel (Nms)
    delta_h_rw=[0.00;0.00;0.00]; % total change in angular momentum of reaction wheel (Nms)

    if t>=0.00
        flag=1;
        h_rw_cur=A*(I_RW*w_rw_cur); 
        delta_h_rw=A*(I_RW*delta_w_rw);

        Td_temp=[0;Td_max*sin(t)]; %Disturbance torque in inertial frame changing with time 
        %frame conversion from inertial frame to body frame
        Td_temp=quatmultiply(quatmultiply(q_sat_cur,Td_temp,flag),[q_sat_cur(1,1);-1*q_sat_cur(2,1);-1*q_sat_cur(3,1);-1*q_sat_cur(4,1)],flag);
        Td=[Td_temp(2,1);Td_temp(3,1);Td_temp(4,1)]; %distuarbance torque in body frame

        for k = 0:h:step
            % Compute h_rw
            h_rw = h_rw_cur + k * delta_h_rw;
    
            % RK4 method for angular velocity
            a = funcEval_dwdt(I_SAT, Iinv, Tc, Td, w_sat_cur, h_rw, h,flag);
            temp = w_sat_cur + a / 2;
    
            b = funcEval_dwdt(I_SAT, Iinv, Tc, Td, temp, h_rw, h,flag);
            temp = w_sat_cur + b / 2;
    
            c = funcEval_dwdt(I_SAT, Iinv, Tc, Td, temp, h_rw, h,flag);
            temp = w_sat_cur + c;
    
            d = funcEval_dwdt(I_SAT, Iinv, Tc, Td, temp, h_rw, h,flag);
    
            w_sat_cur = w_sat_cur + (a / 6 + b / 3 + c / 3 + d / 6);
    
            % RK4 method for quaternion
            w_sat_cur_quat = [0;w_sat_cur];
    
            k1 = qb2i(q_sat_cur, w_sat_cur_quat, h,flag);
            temp2 = q_sat_cur + k1 / 2;
    
            k2 = qb2i(temp2, w_sat_cur_quat, h,flag);
            temp2 = q_sat_cur + k2 / 2;
    
            k3 = qb2i(temp2, w_sat_cur_quat, h,flag);
            temp2 = q_sat_cur + k3;
    
            k4 = qb2i(temp2, w_sat_cur_quat, h,flag);
    
            q_sat_cur = q_sat_cur + (k1/6 + k2/3 + k3/3 + k4/6);
            q_sat_cur=q_sat_cur/((q_sat_cur(1,1)^2+q_sat_cur(2,1)^2+q_sat_cur(3,1)^2+q_sat_cur(4,1)^2)^0.5);
        end

        t_calc=t+step;
        q_sat_calc=q_sat_cur;
        w_sat_calc=w_sat_cur;
        w_rw_calc=w_rw_cur+delta_w_rw;
        h_rw_calc=A*(I_RW*w_rw_calc); 
        h_sat_calc=I_SAT*w_sat_calc;
        h_tot=h_rw_calc+h_sat_calc;
        

    end

end


function w_sat_next = funcEval_dwdt(I_SAT, Iinv, Tc, Td, w_sat_cur, h_rw_cur,h,flag)
    w_sat_next=[0;0;0]; %initialized, compilation error

    if flag==1
        H = (I_SAT * w_sat_cur) + (h_rw_cur); %total angular momentum of satellite + reaction wheel 
        d = cross(w_sat_cur, H);
        T = Tc + Td - d;
        w_sat_next = Iinv * T * h;
    end
end

function q = qb2i(y, w, h,flag)
    q=[1;0;0;0];%initialized, compilation error

    if flag==1
        % Quaternion update based on angular velocity
        q = quatmultiply(w, y,flag) * (h/2);
    end
end

function q = quatmultiply(q1, q2,flag)
    q=[1;0;0;0];%initialized, compilation error

    if flag==1
        % Multiply two quaternions
        q(1,1) = q1(1)*q2(1) - q1(2)*q2(2) - q1(3)*q2(3) - q1(4)*q2(4);
        q(2,1) = q1(1)*q2(2) + q1(2)*q2(1) - q1(3)*q2(4) + q1(4)*q2(3);
        q(3,1) = q1(1)*q2(3) + q1(2)*q2(4) + q1(3)*q2(1) - q1(4)*q2(2);
        q(4,1) = q1(1)*q2(4) - q1(2)*q2(3) + q1(3)*q2(2) + q1(4)*q2(1);
    end
end

== matlab function ADCS/Onboard_temp/Input/MATLAB Function2 ==
  data: duration input; t_calc input; w_sat_cur output; q_sat_cur output; w_rw_cur output; q_sat_i input; q_sat_calc input; w_sat_i input; w_sat_calc input; w_rw_i input; t output; w_rw_calc input
function [w_sat_cur, q_sat_cur,w_rw_cur, t] = variable_time(duration,t_calc,q_sat_i,q_sat_calc, w_sat_i, w_sat_calc,w_rw_i, w_rw_calc)
    %Output initialized
    t=0.00;
    w_sat_cur=w_sat_i; %inital angular vel of satellite rad/s
    q_sat_cur=q_sat_i; %inital attitude of satellite 
    w_rw_cur=w_rw_i; %inital angular vel of reaction wheels rad/s

    if t_calc>0.00 && t_calc<=duration
        t=t_calc; %current time, output from rk4 progation function
        w_sat_cur=w_sat_calc;%current angular vel of satellite (rad/s), output from rk4 progation function
        q_sat_cur=q_sat_calc;%current attitude of satellite, output from rk4 progation function
        w_rw_cur=w_rw_calc;%current angular vel of reaction wheels (rad/s), output from rk4 progation function
    end

end

== matlab function ADCS/Onboard_temp/Onboard_actual/RW torque lim ==
  data: Ti_ini input; Ti_lim output; max_t_rw input
function Ti_lim = Torque_lim(Ti_ini,max_t_rw)
    Ti_lim=Ti_ini;
    for i=1:1:4
        if Ti_ini(i,1)>max_t_rw
            Ti_lim(i,1)=max_t_rw;
        
        elseif Ti_ini(i,1)<(-max_t_rw)
            Ti_lim(i,1)=-max_t_rw;
        
        end
    end   

end
